simulink model "DYN_03x"  (R2021a)
settings: Solver=FixedStepAuto  StartTime=0.0  StopTime=30  FixedStep=0.01  RelTol=1e-3
(part 1 of 14)
settings Model: Creator=TMP  LastModifiedBy=TMP
settings SolverCC: AlgebraicLoopSolver=TrustRegion
settings DebuggingCC: SFMachineParentedDataDiag=warning  ArithmeticOperatorsInVariantConditions=warning
settings SFSimCC: CustomCodeUndefinedFunction=UseInterfaceOnly

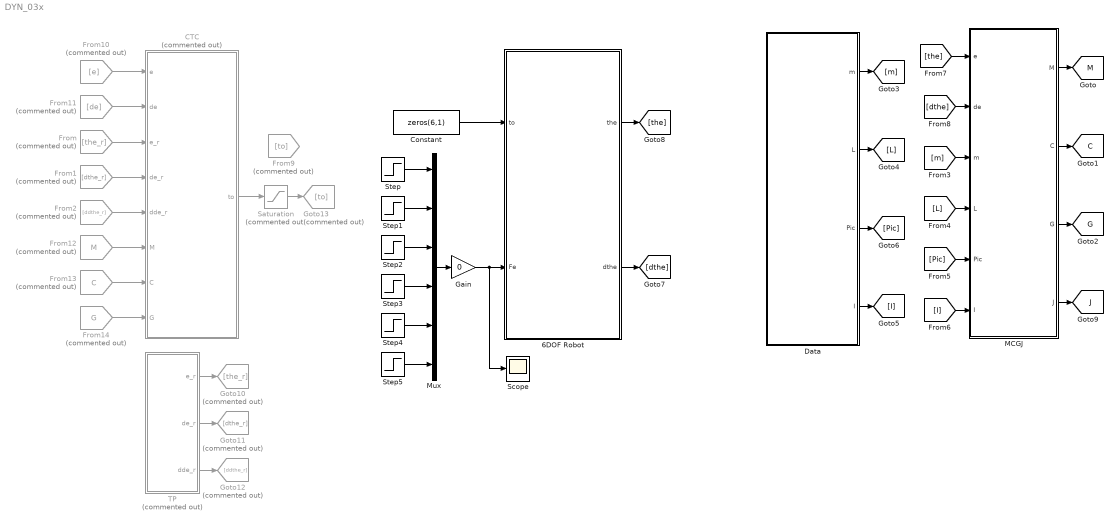
== system DYN_03x ==
  6DOF Robot : Subsystem
  CTC : MATLAB Function  Commented=on  TreatAsAtomicUnit=on
  Constant : Constant  Value=zeros(6,1)
  Data : MATLAB Function  TreatAsAtomicUnit=on
  From : From  Commented=on  GotoTag=the_r
  From1 : From  Commented=on  GotoTag=dthe_r
  From10 : From  Commented=on  GotoTag=e
  From11 : From  Commented=on  GotoTag=de
  From12 : From  Commented=on  GotoTag=M
  From13 : From  Commented=on  GotoTag=C
  From14 : From  Commented=on  GotoTag=G
  From2 : From  Commented=on  GotoTag=ddthe_r
  From9 : From  Commented=on  GotoTag=to
  Gain : Gain  Gain=0
  Goto10 : Goto  Commented=on  GotoTag=the_r
  Goto11 : Goto  Commented=on  GotoTag=dthe_r
  Goto12 : Goto  Commented=on  GotoTag=ddthe_r
  Goto13 : Goto  Commented=on  GotoTag=to
  MCGJ : MATLAB Function  TreatAsAtomicUnit=on
  Mux : Mux  Inputs=6
  Saturation : Saturate  Commented=on  UpperLimit=500  LowerLimit=-500
  Scope : Scope
  Step{,1..5} (6 alike) : Step  Time=10  After=8  SampleTime=0
  TP : Subsystem  Commented=on
  tag scope: C=global, G=global, J=global, M=global
  wires:
  MCGJ/1(M) -> [M]
  MCGJ/2(C) -> [C]
  MCGJ/3(G) -> [G]
  Data/1(m) -> [m]
  Data/2(L) -> [L]
  Data/3(Pic) -> [Pic]
  Data/4(I) -> [I]
  [L] -> MCGJ/4(L)
  [Pic] -> MCGJ/5(Pic)
  [I] -> MCGJ/6(I)
  [m] -> MCGJ/3(m)
  [dthe] -> MCGJ/2(de)
  [the] -> MCGJ/1(e)
  MCGJ/4(J) -> [J]
  6DOF Robot/1(the) -> [the]
  6DOF Robot/2(dthe) -> [dthe]
  Step/1 -> Mux/1
  Step1/1 -> Mux/2
  Step2/1 -> Mux/3
  Step3/1 -> Mux/4
  Step4/1 -> Mux/5
  Step5/1 -> Mux/6
  Mux/1 -> Gain/1
  TP/1(e_r) -> Goto10/1
  TP/2(de_r) -> Goto11/1
  TP/3(dde_r) -> Goto12/1
  From10/1 -> CTC/1(e)
  From11/1 -> CTC/2(de)
  From/1 -> CTC/3(e_r)
  From1/1 -> CTC/4(de_r)
  From2/1 -> CTC/5(dde_r)
  From12/1 -> CTC/6(M)
  From13/1 -> CTC/7(C)
  From14/1 -> CTC/8(G)
  CTC/1(to) -> Saturation/1
  Saturation/1 -> Goto13/1
  Constant/1 -> 6DOF Robot/1(to)
  Gain/1 -> Scope/1, 6DOF Robot/2(Fe)

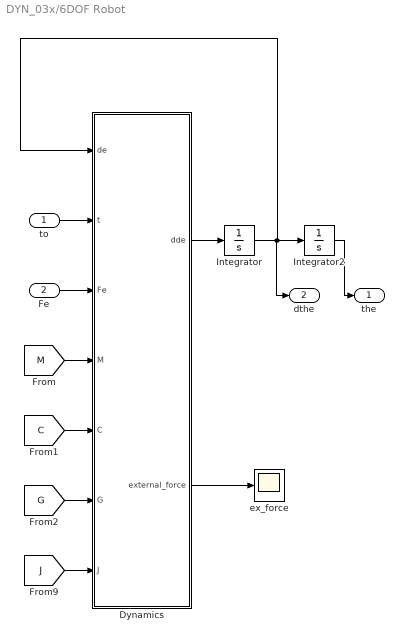
== system DYN_03x/6DOF Robot ==
  to : Inport
  Fe : Inport  Port=2
  Dynamics : MATLAB Function  TreatAsAtomicUnit=on
  Integrator : Integrator  InitialCondition=[pi/6;pi/6;pi/6;pi/6;pi/6;pi/6]  UpperSaturationLimit=pi  LowerSaturationLimit=-pi
  Integrator2 : Integrator  InitialCondition=[pi/6;pi/6;pi/6;pi/6;pi/6;pi/6]  UpperSaturationLimit=[170;120;90;120;60;180]*pi/180  LowerSaturationLimit=-[170;120;90;120;60;180]*pi/180
  ex_force : Scope
  the : Outport  VectorParamsAs1DForOutWhenUnconnected=off
  dthe : Outport  Port=2  VectorParamsAs1DForOutWhenUnconnected=off
  wires:
  Integrator2/1 -> the/1
  Dynamics/1(dde) -> Integrator/1
  [C] -> Dynamics/5(C)
  [J] -> Dynamics/7(J)
  Integrator/1 -> dthe/1, Dynamics/1(de), Integrator2/1
  [M] -> Dynamics/4(M)
  [G] -> Dynamics/6(G)
  to/1 -> Dynamics/2(t)
  Dynamics/2(external_force) -> ex_force/1
  Fe/1 -> Dynamics/3(Fe)

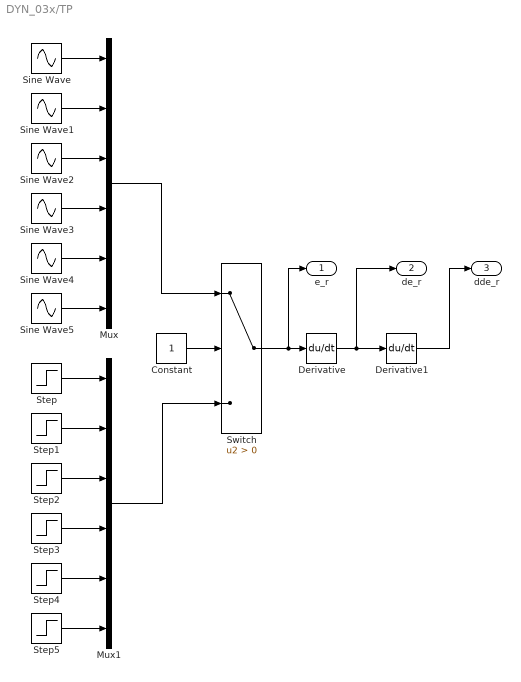
== system DYN_03x/TP ==
  Constant : Constant
  Derivative : Derivative
  Derivative1 : Derivative
  Mux : Mux  Inputs=6
  Mux1 : Mux  Inputs=6
  Sine Wave{,1..5} (6 alike) : Sin  Amplitude=pi/6  Frequency=2*pi*0.2  SampleTime=0
  Step{,1..5} (6 alike) : Step  After=pi/6  SampleTime=0
  Switch : Switch  Criteria=u2 > Threshold
  e_r : Outport  VectorParamsAs1DForOutWhenUnconnected=off
  de_r : Outport  Port=2  VectorParamsAs1DForOutWhenUnconnected=off
  dde_r : Outport  Port=3  VectorParamsAs1DForOutWhenUnconnected=off
  wires:
  Sine Wave/1 -> Mux/1
  Sine Wave1/1 -> Mux/2
  Sine Wave2/1 -> Mux/3
  Sine Wave3/1 -> Mux/4
  Sine Wave4/1 -> Mux/5
  Sine Wave5/1 -> Mux/6
  Mux/1 -> Switch/1
  Constant/1 -> Switch/2
  Mux1/1 -> Switch/3
  Step2/1 -> Mux1/3
  Step5/1 -> Mux1/6
  Step1/1 -> Mux1/2
  Step3/1 -> Mux1/4
  Step/1 -> Mux1/1
  Step4/1 -> Mux1/5
  Switch/1 -> e_r/1, Derivative/1
  Derivative/1 -> de_r/1, Derivative1/1
  Derivative1/1 -> dde_r/1

== matlab function DYN_03x/6DOF Robot/Dynamics ==
  data: de input; t input; Fe input; M input; dde output; C input; G input; J input; external_force output
function [dde,external_force] = DYN_6DOF(de,t,Fe,M,C,G,J)
%%
Fc = diag([0,0,0,0,0,0]);
Fv = 10* diag([1,1,1,1,1,1]);
external_force = Fc*sign(de) + Fv*de + J.'*Fe;
%%
dde = inv(M)*(t - C*de - G - external_force);
